simulink model "SolarCellFinalConstantparameters"  (R2023a)
settings: Solver=VariableStepAuto  StartTime=0.0  StopTime=10.0  RelTol=1e-3
undefined symbols (not defined in the file): Is, Tnom
libraries: spspowerguiLib x1, simulink x1
settings Model: Creator=hp  LastModifiedBy=ask
settings SolverCC: AlgebraicLoopSolver=TrustRegion
settings DataIOCC: ReturnWorkspaceOutputs=off
settings DebuggingCC: UnconnectedInputMsg=warning  UnconnectedOutputMsg=warning  UnconnectedLineMsg=warning  ArithmeticOperatorsInVariantConditions=warning
settings ModelReferenceCC: EnableRefExpFcnMdlSchedulingChecks=on
settings SFSimCC: SimUseLocalCustomCode=off  CustomCodeUndefinedFunction=UseInterfaceOnly
settings RTWCC: RTWUseLocalCustomCode=off
settings CodeAppCC: StateflowObjectComments=on
settings SimscapeCC: SimscapeNormalizeSystem=off

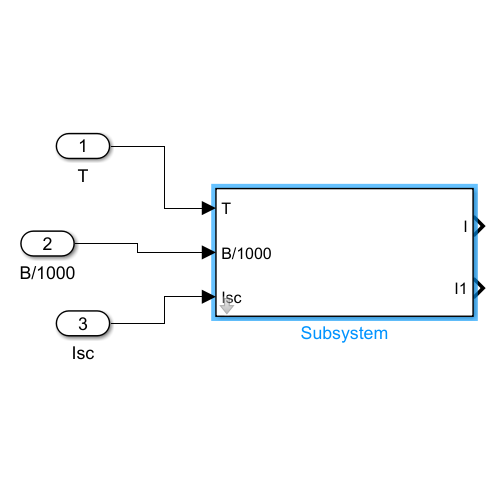
[thumbnail: Simulink's stored preview of the top-level diagram]
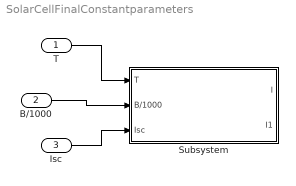
== system SolarCellFinalConstantparameters ==
  T : Inport
  B/1000 : Inport  Port=2
  Isc : Inport  Port=3
  Subsystem : Subsystem  mask{Ns=2, Np=2}
      mask init:
      | N = 1.5;
      | K = 1.3806e-23;
      | q = 1.602e-19;
      | T = 300;
      | Eg = 1;
      | V = 1;
      | vt = 1;
  wires:
  T/1 -> Subsystem/1(T)
  B/1000/1 -> Subsystem/2(B/1000)
  Isc/1 -> Subsystem/3("Isc ")

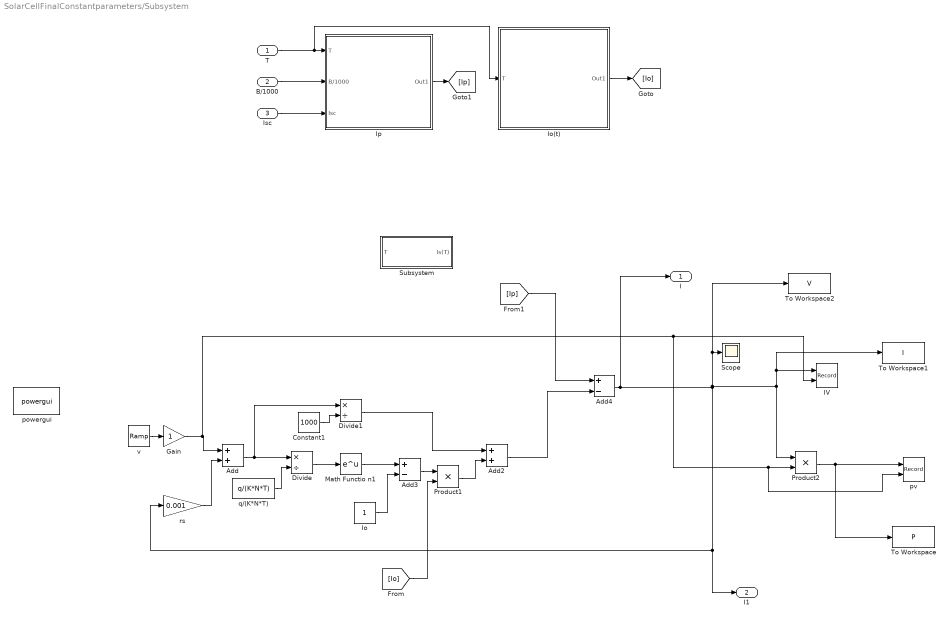
== system SolarCellFinalConstantparameters/Subsystem ==
  T : Inport
  B/1000 : Inport  Port=2
  "Isc " : Inport  Port=3
  Add : Sum
  Add2 : Sum
  Add3 : Sum  Inputs=+-
  Add4 : Sum  Inputs=+-
  Constant1 : Constant  Value=1000
  Divide : Product  Inputs=*/
  Divide1 : Product  Inputs=*/
  Gain : Gain
  "IV " : Record  FileSettingsInternal="{\"entries\":[{\"content\":{\"excelSettings\":{\"content\":{},\"type\":\"Streamout.ExcelSettings\"}},\"type\":\"Streamout.FileSettingStorage\",\"uuid\":\"7bb48b70-b2c6-4921-aca4-abf7892f79b7\"}],\"packageUris\":[\"http://schema.mathworks.com/mf0/streamout_blocks/R2020a\"],\"version\":\"1.0\"}"  Layout=[1 1]  SignalsInternal="{\"entries\":[{\"content\":{\"signals\":[{\"content\":{\"blockPath\":[\"SolarCellFinal/Subsystem/IV  \"],\"dimensions\":[1],\"domain\":\"SolarCellFinal/Subsystem/IV  \",\"lineColor\":\"#a2142f\",\"plots\":[1],\"port\":1,\"signalID\":1217,\"signalName\":\"XY Graph:1\"},\"type\":\"RecordBlkView.Signal\",\"uuid\":\"d5883c97-21e6-4a98-bf2e-33f162b625af\"},{\"content\":{\"blockPath\":[\"SolarCellFinal/Subsystem/IV  \"],\"dimensions\":[1],\"domain\":\"SolarCellFinal/Subsystem/IV  \",\"lineColor\":\"#139fff\",\"plots\":[1],\"port\":2,\"signalID\":1220,\"signalName\":\"XY Graph:2\"},\"type\":\"RecordBlkView.Signal\",\"uuid\":\"afe7445b-ca7b-4c1f-89dc-027bd54b14cd\"}]},\"type\":\"RecordBlkView.InputSignals\",\"uuid\":\"5d828dca-3651-446f-a48f-a21a5ef8b2f5\"}],\"packageUris\":[\"http://schema.mathworks.com/mf0/streamout_blocks/R2020a\"],\"version\":\"1.0\"}"  VisualizationBindings="{\"xyplotplugin\":{\"info\":[{\"series\":[{\"bindingParametersList\":[{\"parameter\":\"X-Axis\",\"signalID\":1217,\"signalName\":\"XY Graph:1\"},{\"parameter\":\"Y-Axis\",\"signalID\":1220,\"signalName\":\"XY Graph:2\"}],\"seriesID\":36507}],\"subplotID\":1}]}}"  CompatibilityTag=XY  st=-1
  Io : Constant
  "Io(t) " : Subsystem
  Ip : Subsystem
  Math Functio n1 : Math  SignedPower=on
  Product1 : Product
  Product2 : Product
  Scope : Scope
  Subsystem : Subsystem
  To Workspace : ToWorkspace  VariableName=P  SaveFormat=Timeseries  SampleTime=-1
  To Workspace1 : ToWorkspace  VariableName=I  SaveFormat=Timeseries  SampleTime=-1
  To Workspace2 : ToWorkspace  VariableName=V  SaveFormat=Timeseries  SampleTime=-1
  powergui : spspowerguiLib/powergui  Priority=1  SimulationMode=Discrete  SampleTime=50e-6  frequency=60  Iterations=50  frequencyindice=0  Pbase=100e6  ErrMax=1e-4  UnitsV=kV  UnitsW=MW  buscounter=0  FunctionMessages=off  echomessages=off  EnableUseOfTLC=off  CurrentSourceSwitches=off  DisableSnubberDevices=off  DisableRonSwitches=off  DisableVfSwitches=off  DisplayEquations=off  AutomaticDiscreteSolvers=off  SolverType=Tustin/Backward Euler (TBE)  Interpol=off  ExternalGateDelay=off  methode=off  Ts=10  x0status=blocks  SPID=off  SwTol=0  HookPort=off  NonlinearTolerance=1e-4  nMaxIteration=100  ContinueOnMaxIteration=off  RestoreLinks=warning  ResistiveCurrentMeasurement=off  Frange=[0:2:500]  Ylog=off  Xlog=on  ShowGrid=off  save=off  variable=ZData  structure=0  ZoomFFT=off  StartTime=0.0  cycles=1  DisplayStyle=1  fundamental=60  FreqAxis=off  MaxFrequency=1000  frequencyindicesteady=1  RmsSteady=1  display=off
  pv : Record  FileSettingsInternal="{\"entries\":[{\"content\":{\"excelSettings\":{\"content\":{},\"type\":\"Streamout.ExcelSettings\"}},\"type\":\"Streamout.FileSettingStorage\",\"uuid\":\"228870c5-18b0-440b-a3b3-3cde1839b402\"}],\"packageUris\":[\"http://schema.mathworks.com/mf0/streamout_blocks/R2020a\"],\"version\":\"1.0\"}"  Layout=[1 1]  SignalsInternal="{\"entries\":[{\"content\":{\"signals\":[{\"content\":{\"blockPath\":[\"SolarCellFinal/Subsystem/pv\"],\"dimensions\":[1],\"domain\":\"SolarCellFinal/Subsystem/pv\",\"lineColor\":\"#a2142f\",\"plots\":[1],\"port\":1,\"signalID\":1209,\"signalName\":\"XY Graph:1\"},\"type\":\"RecordBlkView.Signal\",\"uuid\":\"35ccec0a-e8c1-4c7c-a478-6b19df6d00e6\"},{\"content\":{\"blockPath\":[\"SolarCellFinal/Subsystem/pv\"],\"dimensions\":[1],\"domain\":\"SolarCellFinal/Subsystem/pv\",\"lineColor\":\"#139fff\",\"plots\":[1],\"port\":2,\"signalID\":1212,\"signalName\":\"XY Graph:2\"},\"type\":\"RecordBlkView.Signal\",\"uuid\":\"17ca5639-7dd6-40e9-9712-e7c7e306869b\"}]},\"type\":\"RecordBlkView.InputSignals\",\"uuid\":\"226d1265-d29d-4f70-a508-ada3de9daf5b\"}],\"packageUris\":[\"http://schema.mathworks.com/mf0/streamout_blocks/R2020a\"],\"version\":\"1.0\"}"  VisualizationBindings="{\"xyplotplugin\":{\"info\":[{\"series\":[{\"bindingParametersList\":[{\"parameter\":\"X-Axis\",\"signalID\":1209,\"signalName\":\"XY Graph:1\"},{\"parameter\":\"Y-Axis\",\"signalID\":1212,\"signalName\":\"XY Graph:2\"}],\"seriesID\":64578}],\"subplotID\":1}]}}"  CompatibilityTag=XY  st=-1
  q/(K*N*T) : Constant  Value=q/(K*N*T)
  "rs " : Gain  Gain=0.001
  v : simulink/Sources/Ramp  slope=30  start=0  InitialOutput=0
  I : Outport
  I1 : Outport  Port=2
  wires:
  v/1 -> Gain/1
  Gain/1 -> pv/2, Product2/2, "IV "/2, Add/1
  "rs "/1 -> Add/2
  Add/1 -> Divide1/1, Divide/1
  q/(K*N*T)/1 -> Divide/2
  Divide/1 -> Math Functio n1/1
  Math Functio n1/1 -> Add3/1
  Io/1 -> Add3/2
  Constant1/1 -> Divide1/2
  Add3/1 -> Product1/1
  [Io] -> Product1/2
  Product1/1 -> Add2/2
  Divide1/1 -> Add2/1
  Add2/1 -> Add4/2
  [Ip] -> Add4/1
  Add4/1 -> I/1, "IV "/1, To Workspace1/1, Product2/1, To Workspace2/1, Scope/1, I1/1, "rs "/1
  "Io(t) "/1(Out1) -> [Io]
  Ip/1(Out1) -> [Ip]
  B/1000/1 -> Ip/2(B/1000)
  "Isc "/1 -> Ip/3("Isc ")
  T/1 -> "Io(t) "/1("T "), Ip/1(T)
  Product2/1 -> To Workspace/1, pv/1

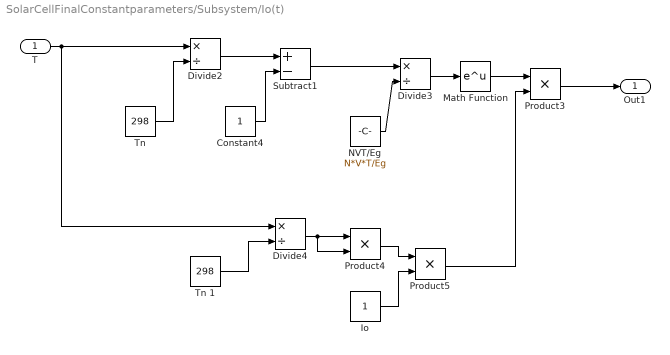
== system SolarCellFinalConstantparameters/Subsystem/Io(t)  ==
  "T " : Inport
  Constant4 : Constant
  Divide2 : Product  Inputs=*/
  Divide3 : Product  Inputs=*/
  Divide4 : Product  Inputs=*/
  "Io " : Constant
  Math Function : Math  SignedPower=on
  NVT/Eg : Constant  Value=N*V*T/Eg
  Product3 : Product
  Product4 : Product
  Product5 : Product
  Subtract1 : Sum  Inputs=+-
  "Tn " : Constant  Value=298
  Tn 1 : Constant  Value=298
  Out1 : Outport
  wires:
  Divide2/1 -> Subtract1/1
  "Io "/1 -> Product5/2
  Math Function/1 -> Product3/1
  Product4/1 -> Product5/1
  Divide4/1 -> Product4/2, Product4/1
  Constant4/1 -> Subtract1/2
  "Tn "/1 -> Divide2/2
  NVT/Eg/1 -> Divide3/2
  Divide3/1 -> Math Function/1
  Subtract1/1 -> Divide3/1
  Product5/1 -> Product3/2
  Tn 1/1 -> Divide4/2
  Product3/1 -> Out1/1
  "T "/1 -> Divide4/1, Divide2/1

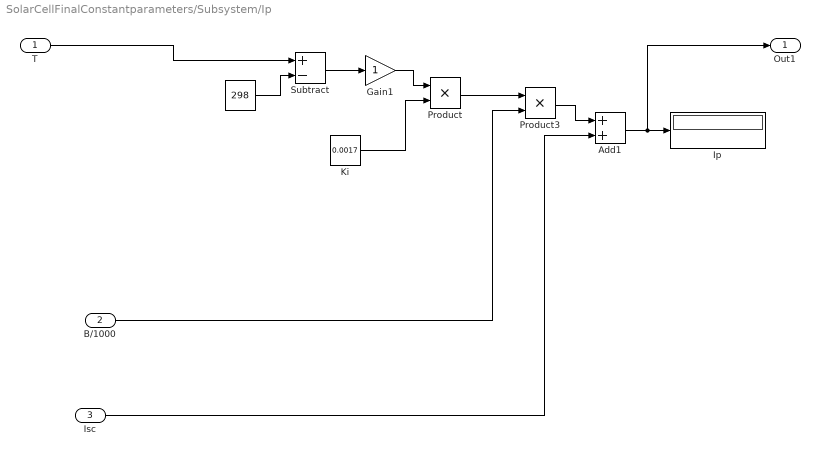
== system SolarCellFinalConstantparameters/Subsystem/Ip ==
  T : Inport
  B/1000 : Inport  Port=2
  "Isc " : Inport  Port=3
  " " : Constant  Value=298
  Add1 : Sum
  Gain1 : Gain
  "Ip " : Display
  "Ki " : Constant  Value=0.0017
  Product : Product
  Product3 : Product
  Subtract : Sum  Inputs=+-
  Out1 : Outport
  wires:
  T/1 -> Subtract/1
  Subtract/1 -> Gain1/1
  Product3/1 -> Add1/1
  Product/1 -> Product3/1
  Gain1/1 -> Product/1
  "Isc "/1 -> Add1/2
  B/1000/1 -> Product3/2
  Add1/1 -> Out1/1, "Ip "/1
  "Ki "/1 -> Product/2
  " "/1 -> Subtract/2

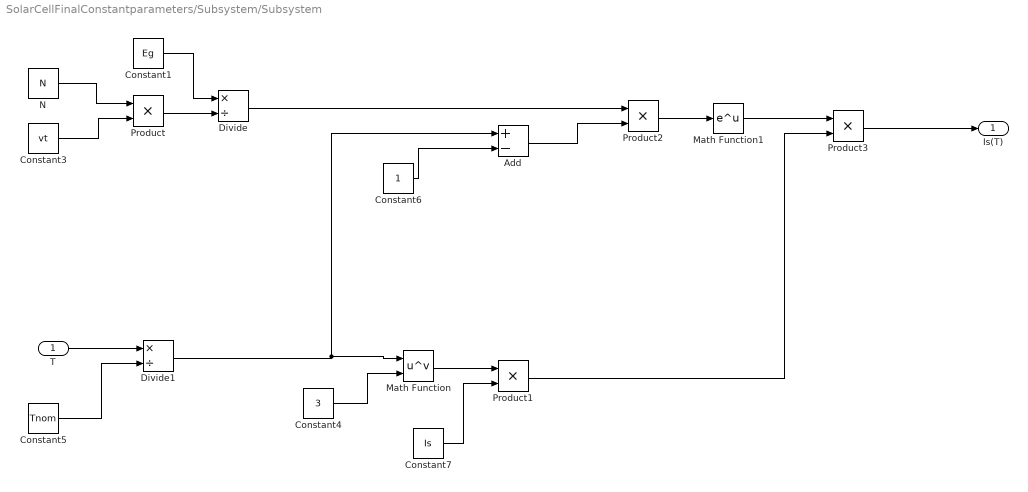
== system SolarCellFinalConstantparameters/Subsystem/Subsystem ==
  T : Inport
  Add : Sum  Inputs=+-
  Constant1 : Constant  Value=Eg
  Constant3 : Constant  Value=vt
  Constant4 : Constant  Value=3
  Constant5 : Constant  Value=Tnom
  Constant6 : Constant
  Constant7 : Constant  Value=Is
  Divide : Product  Inputs=*/
  Divide1 : Product  Inputs=*/
  Math Function : Math  Operator=pow  SignedPower=on
  Math Function1 : Math  SignedPower=on
  N : Constant  Value=N
  Product{,1..3} (4 alike) : Product
  Is(T) : Outport
  wires:
  Constant1/1 -> Divide/1
  Product/1 -> Divide/2
  N/1 -> Product/1
  Constant3/1 -> Product/2
  Constant6/1 -> Add/2
  Divide1/1 -> Math Function/1, Add/1
  T/1 -> Divide1/1
  Constant5/1 -> Divide1/2
  Constant4/1 -> Math Function/2
  Math Function/1 -> Product1/1
  Constant7/1 -> Product1/2
  Divide/1 -> Product2/1
  Add/1 -> Product2/2
  Product2/1 -> Math Function1/1
  Math Function1/1 -> Product3/1
  Product1/1 -> Product3/2
  Product3/1 -> Is(T)/1
